simulink subsystem "HIL_Send_TCP_Data_6gdl_2021"  (R2021a)
settings: Solver=VariableStepAuto  StartTime=0.0  StopTime=10.0  RelTol=1e-3
model mask{mi_ip=mi_ip, mi_port=mi_port, f=0}
  mask prompts: mi_ip "Server IP"; mi_port "Server Port"; f "Sampling Frequency"
libraries: slrealtimeutilitieslib x2, slrealtimeiplib x1
settings Model: Creator=ramuj  LastModifiedBy=aceao
settings DebuggingCC: UnconnectedInputMsg=none  UnconnectedOutputMsg=none  UnconnectedLineMsg=none
settings ModelReferenceCC: EnableRefExpFcnMdlSchedulingChecks=off
settings RTWCC: Description=Generic Real-Time Target  DLArmComputeVersion=20.02.1

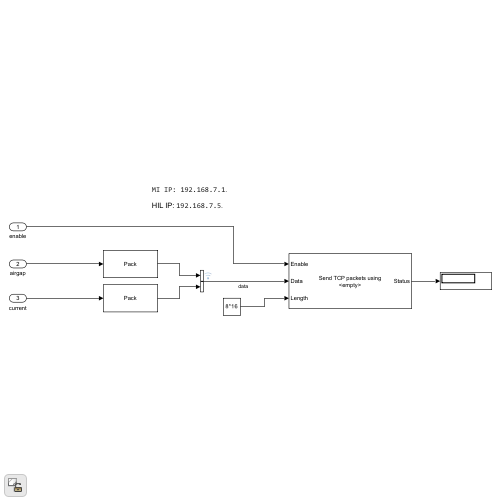
[thumbnail: Simulink's stored preview of the top-level diagram]
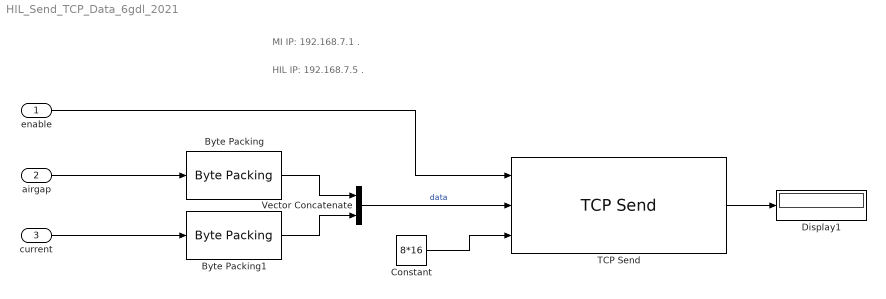
== system HIL_Send_TCP_Data_6gdl_2021 ==
  note: MI IP: 192.168.7.1 .
  note: HIL IP: 192.168.7.5 .
  enable : Inport
  airgap : Inport  Port=2
  current : Inport  Port=3
  Byte Packing : slrealtimeutilitieslib/Byte Packing  MaskPackedDataType=uint8  MaskUnpackedDataTypes={'double'}  MaskAlignment=1
  Byte Packing1 : slrealtimeutilitieslib/Byte Packing  MaskPackedDataType=uint8  MaskUnpackedDataTypes={'double'}  MaskAlignment=1
  Constant : Constant  Value=8*16
  Display1 : Display
  TCP Send : slrealtimeiplib/TCP Send  socketAddPortVal=Client: 0.0.0.0:0  sampleTime=1/f
  Vector Concatenate : Concatenate
  wires:
  TCP Send/1 -> Display1/1
  Byte Packing/1 -> Vector Concatenate/1
  Byte Packing1/1 -> Vector Concatenate/2
  Vector Concatenate/1 -> TCP Send/2  "data"
  Constant/1 -> TCP Send/3
  enable/1 -> TCP Send/1
  current/1 -> Byte Packing1/1
  airgap/1 -> Byte Packing/1
